simulink model "gm_dspmultichannelhdl_fil"  (R2025b)
settings: Solver=FixedStepDiscrete  StartTime=0.0  StopTime=0.5  RelTol=1e-3
InitFcn:
  | Fpass = 0.2; % Passband Frequency
  | Fstop = 0.3; % Stopband Frequency
  | Apass = 1;    % Passband Attenuation (dB)
  | Astop = 60;   % Stopband Attenuation (dB)
  | 
  | f = fdesign.lowpass('Fp,Fst,Ap,Ast',Fpass,Fstop,Apass,Astop);
  | Hlp = design(f, 'equiripple','FilterStructure', 'dffir'); % Lowpass
  | Numerator = Hlp.Numerator;  % coefficients of lowpass filter
libraries: dspsrcs4 x2, simulink x1, fillib x1
settings Model: Creator=The MathWorks, Inc.  LastModifiedBy=KoayXianCong
settings SolverCC: AlgebraicLoopSolver=TrustRegion
settings DataIOCC: LimitDataPoints=on  SaveFormat=Array  ReturnWorkspaceOutputs=off
settings OptimizationCC: BlockReduction=off  ConditionallyExecuteInputs=off  DefaultParameterBehavior=Inlined  ExpressionDepthLimit=2147483647.0  LifeSpan=inf  SimCompilerOptimization=on
settings DebuggingCC: AlgebraicLoopMsg=error  UnderspecifiedInitializationDetection=Classic  MergeDetectMultiDrivingBlocksExec=none  SolverPrmCheckMsg=warning  InheritedTsInSrcMsg=none  ParameterPrecisionLossMsg=none  UnconnectedInputMsg=warning  UnconnectedOutputMsg=warning  UnconnectedLineMsg=warning  StateNameClashWarn=warning  SymbolicDimsDataTypeCodeGenerationDiagnostic=none  SFUnexpectedBacktrackingDiag=warning  SFNoUnconditionalDefaultTransitionDiag=warning  SFExecutionAtInitializationDiag=none  ArithmeticOperatorsInVariantConditions=warning
settings HardwareCC: ProdBitPerPointer=32.0  ProdBitPerSizeT=32.0  ProdBitPerPtrDiffT=32.0  ProdLargestAtomicFloat=None  ProdIntDivRoundTo=Undefined  ProdEndianess=Unspecified  ProdWordSize=32.0  ProdHWDeviceType=ASIC/FPGA->ASIC/FPGA  TargetBitPerPointer=64.0  TargetBitPerSizeT=64.0  TargetBitPerPtrDiffT=64.0  TargetLongLongMode=on  TargetIntDivRoundTo=Zero  TargetEndianess=LittleEndian  TargetWordSize=64.0  TargetHWDeviceType=Generic->MATLAB Host Computer  ProdEqTarget=off
settings ModelReferenceCC: EnableRefExpFcnMdlSchedulingChecks=on  PropagateSignalLabelsOutOfModel=off
settings SFSimCC: SimUseLocalCustomCode=off  CustomCodeUndefinedFunction=UseInterfaceOnly
settings RTWCC: RTWUseLocalCustomCode=off  GPUComputeCapability=3.5
settings CodeAppCC: StateflowObjectComments=on
settings GRTTargetCC: TargetLangStandard=C89/C90 (ANSI)
settings ConfigComp: CovMetricSettings=dw  CovSaveCumulativeToWorkspaceVar=on  CovSaveSingleToWorkspaceVar=on  CovExternalEMLEnable=off

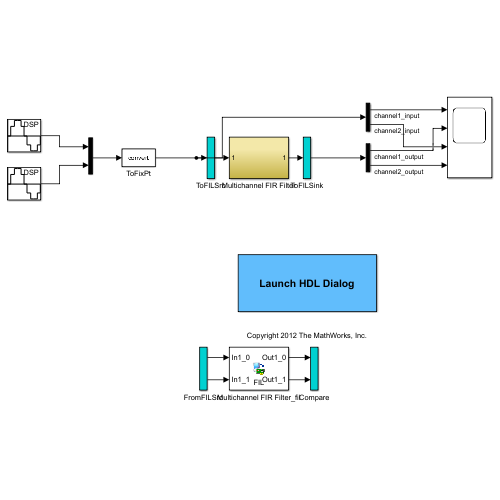
[thumbnail: Simulink's stored preview of the top-level diagram]
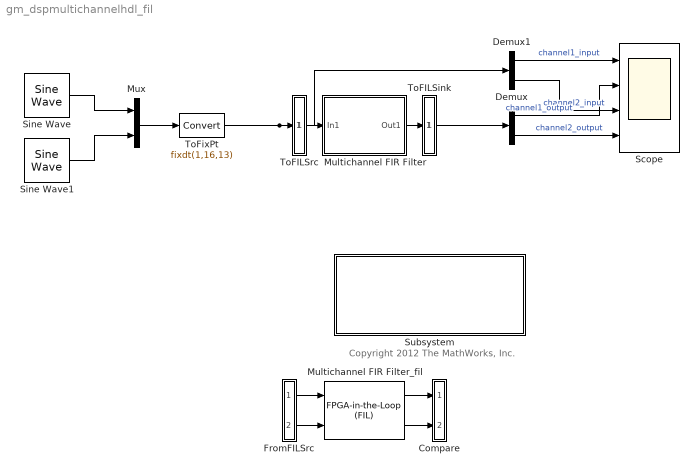
== system gm_dspmultichannelhdl_fil ==
  note: Copyright 2012 The MathWorks, Inc.
  Compare : Subsystem
      mask Display: disp('')
  Demux : Demux  Outputs=2
  Demux1 : Demux  Outputs=2
  FromFILSrc : Subsystem
      mask Display: disp('')
  Multichannel FIR Filter : Subsystem
  Multichannel FIR Filter_fil : fillib/FPGA-in-the-Loop (FIL)  ForceInterfaceUpdate=0.65011
  Mux : Mux  Inputs=2
  Scope : Scope  NumInputPorts=4
      settings: TimeSpan=0.5  ActiveDisplayYMinimum=-1  ActiveDisplayYMaximum=1
  Sine Wave : dspsrcs4/Sine Wave  Amplitude=1  Frequency=100  Phase=0  SampleMode=Discrete  OutComplex=Real  CompMethod=Trigonometric fcn  TableSize=Speed  SampleTime=1/2000  SamplesPerFrame=1  ResetState=Restart at time zero  OutputFrames=on  dataType=double  wordLen=16  udDataType=sfix(16)  fracBitsMode=Best precision  numFracBits=15  OutDataTypeStr=double  LastOutDataTypeStr=double
  Sine Wave1 : dspsrcs4/Sine Wave  Amplitude=1  Frequency=400  Phase=0  SampleMode=Discrete  OutComplex=Real  CompMethod=Trigonometric fcn  TableSize=Speed  SampleTime=1/2000  SamplesPerFrame=1  ResetState=Restart at time zero  OutputFrames=on  dataType=double  wordLen=16  udDataType=sfix(16)  fracBitsMode=Best precision  numFracBits=15  OutDataTypeStr=double  LastOutDataTypeStr=double
  Subsystem : Subsystem
      settings: OpenFcn=hdldialog(bdroot)
      mask Display: disp('Launch HDL Dialog')
  ToFILSink : Subsystem
      mask Display: disp('')
  ToFILSrc : Subsystem
      mask Display: disp('')
  ToFixPt : DataTypeConversion  OutDataTypeStr=fixdt(1,16,13)  SaturateOnIntegerOverflow=off  RndMeth=Floor
  wires:
  Mux/1 -> ToFixPt/1
  Sine Wave/1 -> Mux/1
  Demux1/1 -> Scope/1  "channel1_input"
  Demux1/2 -> Scope/3  "channel2_input"
  Demux/2 -> Scope/4  "channel2_output"
  ToFixPt/1 -> Demux1/1, ToFILSrc/1(in1)
  Sine Wave1/1 -> Mux/2
  Demux/1 -> Scope/2  "channel1_output"
  ToFILSrc/1(out1) -> Multichannel FIR Filter/1(In1)
  Multichannel FIR Filter/1(Out1) -> ToFILSink/1(in1)
  ToFILSink/1(out1) -> Demux/1
  FromFILSrc/1(out1) -> Multichannel FIR Filter_fil/1
  FromFILSrc/2(out2) -> Multichannel FIR Filter_fil/2
  Multichannel FIR Filter_fil/1 -> Compare/1(in1)
  Multichannel FIR Filter_fil/2 -> Compare/2(in2)

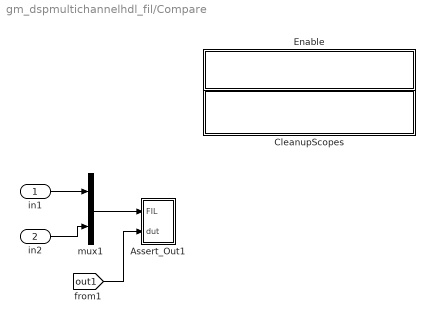
== system gm_dspmultichannelhdl_fil/Compare ==
  in1 : Inport
  in2 : Inport  Port=2
  Assert_Out1 : Subsystem
  CleanupScopes : Subsystem
      settings: OpenFcn=|
      | blkName = gcb; %self block
      | idx = regexp(blkName, '/CleanupScopes$', 'once');
      | blkParent = blkName(1:idx-1);
      | blks=find_system(blkParent, 'LookUnderMasks', 'all','blocktype', 'Scope');
      | for itr = 1:length(blks)
      | 	 hScopeCfg = get_param(blks{itr},'ScopeConfiguration');
      | 	 hScopeCfg.Visible = ~ hScopeCfg.Visible;
      | end
      | drawnow;
      mask Display: fprintf(message('hdlcoder:cosim:vnl_dblclick').getString());
  Enable : Subsystem
      settings: OpenFcn=|
      | blkName = gcb;
      | idx = regexp(blkName, '/Enable$', 'once');
      | blkParent = blkName(1:idx-1);
      | blks=find_system(blkParent, 'LookUnderMasks', 'all','blocktype', 'Assertion');
      | e = get_param(blks{1}, 'Enabled');
      | if strcmp(e, 'on'), f= 'off';, else, f = 'on';, end
      | for ii=1:length(blks), set_param(blks{ii}, 'Enabled', f);, end
      | set_param(gcb, 'MaskDisplay',['fprintf(message(''hdlcoder:cosim:vnl_dblclick_assertions'',','''',upper(e),'''',').getString())']);
      mask Display: fprintf(message('hdlcoder:cosim:vnl_dblclick_assertions','OFF').getString());
  mux1 : Mux  Inputs=2
  wires:
  in1/1 -> mux1/1
  mux1/1 -> Assert_Out1/1(FIL)
  in2/1 -> mux1/2
  [out1] -> Assert_Out1/2(dut)

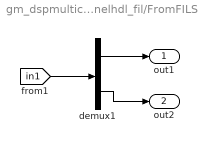
== system gm_dspmultichannelhdl_fil/FromFILSrc ==
  demux1 : Demux  Outputs=2
      settings: DisplayOption=none
  out1 : Outport
  out2 : Outport  Port=2
  wires:
  [in1] -> demux1/1
  demux1/2 -> out2/1
  demux1/1 -> out1/1

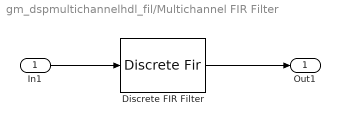
== system gm_dspmultichannelhdl_fil/Multichannel FIR Filter ==
  In1 : Inport
  Discrete FIR Filter : DiscreteFir  FilterStructure=Direct form symmetric  Coefficients=Numerator
  Out1 : Outport  VectorParamsAs1DForOutWhenUnconnected=off
  wires:
  In1/1 -> Discrete FIR Filter/1
  Discrete FIR Filter/1 -> Out1/1

== system gm_dspmultichannelhdl_fil/Subsystem ==

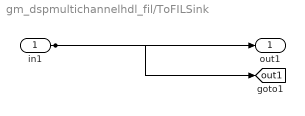
== system gm_dspmultichannelhdl_fil/ToFILSink ==
  in1 : Inport
  out1 : Outport
  tag scope: out1=global
  wires:
  in1/1 -> out1/1, [out1]

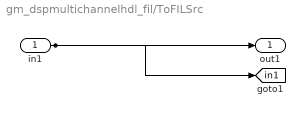
== system gm_dspmultichannelhdl_fil/ToFILSrc ==
  in1 : Inport
  out1 : Outport
  tag scope: in1=global
  wires:
  in1/1 -> out1/1, [in1]

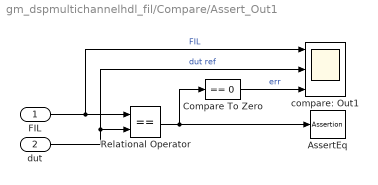
== system gm_dspmultichannelhdl_fil/Compare/Assert_Out1 ==
  FIL : Inport
  dut : Inport  Port=2
  AssertEq : Assertion  StopWhenAssertionFail=off
  Compare To Zero : simulink/Logic and Bit Operations/Compare To Zero  relop===  OutDataTypeStr=boolean
  Relational Operator : RelationalOperator  Operator===  OutDataTypeStr=boolean  InputSameDT=off
  compare: Out1 : Scope  NumInputPorts=3
      settings: ActiveDisplayYMinimum=-5  ActiveDisplayYMaximum=5
  wires:
  Compare To Zero/1 -> compare: Out1/3  "err"
  Relational Operator/1 -> Compare To Zero/1, AssertEq/1
  FIL/1 -> compare: Out1/1, Relational Operator/1  "FIL"
  dut/1 -> compare: Out1/2, Relational Operator/2  "dut ref"

== system gm_dspmultichannelhdl_fil/Compare/CleanupScopes ==

== system gm_dspmultichannelhdl_fil/Compare/Enable ==
